simulink model "simulation"  (R2020b)
settings: Solver=VariableStepAuto  StartTime=0.0  StopTime=60  RelTol=1e-3
settings Model: Creator=block  LastModifiedBy=block

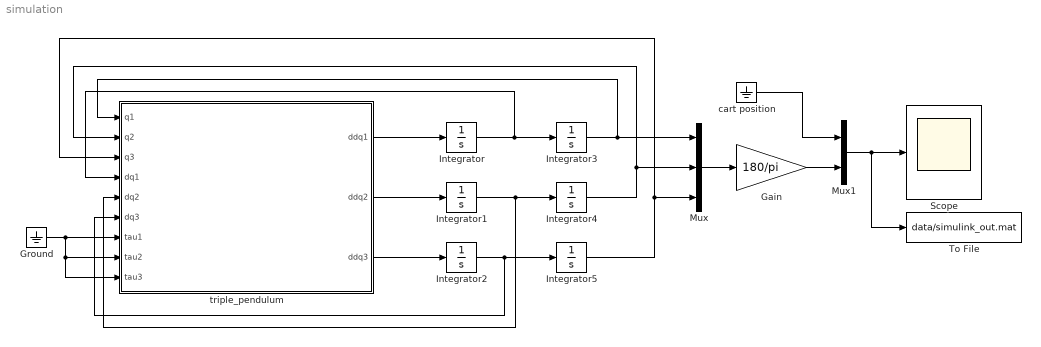
== system simulation ==
  Gain : Gain  Gain=180/pi
  Ground : Ground
  Integrator{,1..2,4..5} (5 alike) : Integrator
  Integrator3 : Integrator  InitialCondition=2.62
  Mux : Mux  Inputs=3
  Mux1 : Mux  Inputs=2
  Scope : Scope
  To File : ToFile  Filename=data/simulink_out.mat  MatrixName=position  SaveFormat=Timeseries  SampleTime=0.01
  cart position : Ground
  triple_pendulum : MATLAB Function  TreatAsAtomicUnit=on
  wires:
  triple_pendulum/1(ddq1) -> Integrator/1
  triple_pendulum/2(ddq2) -> Integrator1/1
  triple_pendulum/3(ddq3) -> Integrator2/1
  Integrator/1 -> triple_pendulum/4(dq1), Integrator3/1
  Integrator1/1 -> triple_pendulum/5(dq2), Integrator4/1
  Integrator2/1 -> triple_pendulum/6(dq3), Integrator5/1
  Integrator3/1 -> Mux/1, triple_pendulum/1(q1)
  Integrator4/1 -> Mux/2, triple_pendulum/2(q2)
  Integrator5/1 -> Mux/3, triple_pendulum/3(q3)
  Ground/1 -> triple_pendulum/9(tau3), triple_pendulum/8(tau2), triple_pendulum/7(tau1)
  Gain/1 -> Mux1/2
  Mux/1 -> Gain/1
  Mux1/1 -> To File/1, Scope/1
  cart position/1 -> Mux1/1

== matlab function simulation/triple_pendulum ==
  data: q1 input; ddq1 output; ddq2 output; ddq3 output; q2 input; q3 input; dq1 input; dq2 input; dq3 input; tau1 input; tau2 input; tau3 input
function [ddq1,ddq2,ddq3] = triple_pendulum(q1,q2,q3,dq1,dq2,dq3,tau1,tau2,tau3)
    ret = ode(q1,q2,q3,dq1,dq2,dq3,tau1,tau2,tau3);
    
    ddq1 = ret(1);
    ddq2 = ret(2);
    ddq3 = ret(3);
end
